simulink model "madar"  (Simulink 7.5)
settings: Solver=ode45  StartTime=0.0  StopTime=24  MaxStep=inf  RelTol=1e-3
values from neighbouring files (symbols this model uses):
  R1 = Req/2    [trans-test.m]
  R2 = (Req/2)*((Vlv/Vhv)^2)    [trans-test.m]
  Rc = Voc^2/Pc    [trans-test.m]
  S = input('enter the power')    [trans-test.m]
  Vhv = input('enter high voltage')    [trans-test.m]
  Vlv = input('enter low voltage')    [trans-test.m]
  X1 = Xeq/2    [trans-test.m]
  X2 = (Xeq/2)*((Vlv/Vhv)^2)    [trans-test.m]
  Xm = Voc/Im    [trans-test.m]
libraries: powerlib x23, powerlib_extras x6
settings Model: Creator=Kian  LastModifiedBy=Kian
settings SolverCC: AutoInsertRateTranBlk=on
settings DataIOCC: OutputSaveName=Iout
settings DebuggingCC: SolverPrmCheckMsg=none

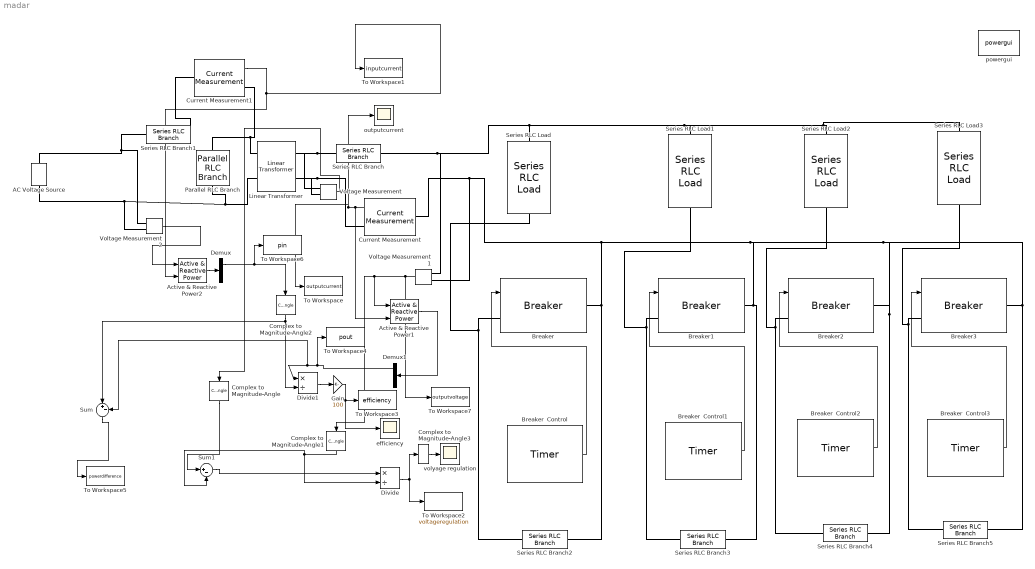
== system madar ==
  AC Voltage Source : powerlib/Electrical Sources/AC Voltage Source  DialogController=POWERSYS.PowerSysDialog  SystemSampleTime=-1  Amplitude=Vhv*(2^.5)  Phase=0  Frequency=50  SampleTime=0  Measurements=None
  Active & Reactive Power1 : powerlib_extras/Measurements/Active & Reactive Power  DialogController=POWERSYS.PowerSysDialog  SystemSampleTime=-1  f1=50
  Active & Reactive Power2 : powerlib_extras/Measurements/Active & Reactive Power  DialogController=POWERSYS.PowerSysDialog  SystemSampleTime=-1  f1=50
  Breaker{,1..3} (4 alike) : powerlib/Elements/Breaker  DialogController=POWERSYS.PowerSysDialog  SystemSampleTime=-1  BreakerResistance=0.000001  InitialState=0  SnubberResistance=inf  SnubberCapacitance=0  SwitchingTimes="[ 1/60  5/60 ]"  External=on  Measurements=None  MoreParameters=off  NoBreakLoop=off
  Breaker  Control : powerlib_extras/Control  Blocks/Timer  DialogController=POWERSYS.PowerSysDialog  SystemSampleTime=-1  t=[0 0.00001 7]  e=[0 1 0 ]
  Breaker  Control1 : powerlib_extras/Control  Blocks/Timer  DialogController=POWERSYS.PowerSysDialog  SystemSampleTime=-1  t=[0 7 12]  e=[0 1 0 ]
  Breaker  Control2 : powerlib_extras/Control  Blocks/Timer  DialogController=POWERSYS.PowerSysDialog  SystemSampleTime=-1  t=[0 12 20]  e=[0 1 0 ]
  Breaker  Control3 : powerlib_extras/Control  Blocks/Timer  DialogController=POWERSYS.PowerSysDialog  SystemSampleTime=-1  t=[0 20 24]  e=[0 1 0 ]
  Complex to Magnitude-Angle{,1..3} (4 alike) : ComplexToMagnitudeAngle  Output=Magnitude
  Current Measurement : powerlib/Measurements/Current Measurement  DialogController=POWERSYS.PowerSysDialog  SystemSampleTime=-1  PhasorSimulation=off  OutputType=Complex  PSBequivalent=0
  Current Measurement1 : powerlib/Measurements/Current Measurement  DialogController=POWERSYS.PowerSysDialog  SystemSampleTime=-1  PhasorSimulation=off  OutputType=Complex  PSBequivalent=0
  Demux : Demux  Outputs=2
  Demux1 : Demux  Outputs=2
  Divide : Product  Inputs=*/  OutDataType=fixdt(1, 16)  OutScaling=2^-10
  Divide1 : Product  Inputs=*/  OutDataType=fixdt(1, 16)  OutScaling=2^-10
  Gain : Gain  Gain=100  ParameterDataType=fixdt(1, 16)  ParameterScaling=2^0  OutDataType=fixdt(1, 16)  OutScaling=2^0
  Linear Transformer : powerlib/Elements/Linear Transformer  DialogController=POWERSYS.PowerSysDialog  PhysicalDomain=powersysdomain  SubClassName=unknown  LeftPortType=p1  RightPortType=p1  LConnTagsString=a|b  RConnTagsString=A|B  UNITS=SI  NominalPower=[ S 50 ]  winding1="[ Vhv  0  0 ]"  winding2="[ Vlv  0  0 ]"  ThreeWindings=off  winding3=[ ]  RmLm=[ 0 0 ]  Measurements=None  DataType=off
  Parallel RLC Branch : powerlib/Elements/Parallel RLC Branch  DialogController=POWERSYS.PowerSysDialog  PhysicalDomain=powersysdomain  SubClassName=unknown  LeftPortType=p1  RightPortType=p1  LConnTagsString=a  RConnTagsString=__new0  BranchType=RL  Resistance=Rc*((Vhv/Vlv)^2)  Inductance=Xm*((Vhv/Vlv)^2)/(100*pi)  SetiL0=off  InitialCurrent=0  Capacitance=0  Setx0=off  InitialVoltage=0  Measurements=None
  Series RLC Branch : powerlib/Elements/Series RLC Branch  DialogController=POWERSYS.PowerSysDialog  PhysicalDomain=powersysdomain  SubClassName=unknown  LeftPortType=p1  RightPortType=p1  LConnTagsString=__new0  RConnTagsString=__new0  BranchType=RL  Resistance=R2  Inductance=X2/(100*pi)  SetiL0=off  InitialCurrent=0  Capacitance=0  Setx0=off  InitialVoltage=0  Measurements=None
  Series RLC Branch1 : powerlib/Elements/Series RLC Branch  DialogController=POWERSYS.PowerSysDialog  PhysicalDomain=powersysdomain  SubClassName=unknown  LeftPortType=p1  RightPortType=p1  LConnTagsString=__new0  RConnTagsString=__new0  BranchType=RL  Resistance=R1  Inductance=X1/(100*pi)  SetiL0=off  InitialCurrent=0  Capacitance=0  Setx0=off  InitialVoltage=0  Measurements=None
  Series RLC Branch{2..5} (4 alike) : powerlib/Elements/Series RLC Branch  DialogController=POWERSYS.PowerSysDialog  PhysicalDomain=powersysdomain  SubClassName=unknown  LeftPortType=p1  RightPortType=p1  LConnTagsString=__new0  RConnTagsString=__new0  BranchType=R  Resistance=1000000  Inductance=X2/(100*pi)  SetiL0=off  InitialCurrent=0  Capacitance=0  Setx0=off  InitialVoltage=0  Measurements=None
  Series RLC Load : powerlib/Elements/Series RLC Load  DialogController=POWERSYS.PowerSysDialog  PhysicalDomain=powersysdomain  SubClassName=unknown  LeftPortType=p1  RightPortType=p1  LConnTagsString=a  RConnTagsString=__new0  NominalVoltage=Vlv  NominalFrequency=50  ActivePower=0.3*S*0.8  InductivePower=0.3*S*0.6  CapacitivePower=0  Setx0=off  InitialVoltage=0  SetiL0=off  InitialCurrent=0  Measurements=None
  Series RLC Load1 : powerlib/Elements/Series RLC Load  DialogController=POWERSYS.PowerSysDialog  PhysicalDomain=powersysdomain  SubClassName=unknown  LeftPortType=p1  RightPortType=p1  LConnTagsString=a  RConnTagsString=__new0  NominalVoltage=Vlv  NominalFrequency=50  ActivePower=0.75*S  InductivePower=0  CapacitivePower=0  Setx0=off  InitialVoltage=0  SetiL0=off  InitialCurrent=0  Measurements=None
  Series RLC Load2 : powerlib/Elements/Series RLC Load  DialogController=POWERSYS.PowerSysDialog  PhysicalDomain=powersysdomain  SubClassName=unknown  LeftPortType=p1  RightPortType=p1  LConnTagsString=a  RConnTagsString=__new0  NominalVoltage=Vlv  NominalFrequency=50  ActivePower=S*0.9  InductivePower=S*0.435  CapacitivePower=0  Setx0=off  InitialVoltage=0  SetiL0=off  InitialCurrent=0  Measurements=None
  Series RLC Load3 : powerlib/Elements/Series RLC Load  DialogController=POWERSYS.PowerSysDialog  PhysicalDomain=powersysdomain  SubClassName=unknown  LeftPortType=p1  RightPortType=p1  LConnTagsString=a  RConnTagsString=__new0  NominalVoltage=Vlv  NominalFrequency=50  ActivePower=0.5*S*0.85  InductivePower=0.5*S*0.526  CapacitivePower=0  Setx0=off  InitialVoltage=0  SetiL0=off  InitialCurrent=0  Measurements=None
  Sum : Sum  Inputs=|+-  OutDataType=fixdt(1, 16)  OutScaling=2^0
  Sum1 : Sum  Inputs=|+-  OutDataType=fixdt(1, 16)  OutScaling=2^0
  To Workspace : ToWorkspace  VariableName=outputcurrent  SampleTime=-1  SaveFormat=Structure With Time
  To Workspace1 : ToWorkspace  VariableName=inputcurrent  SampleTime=-1  SaveFormat=Structure
  To Workspace2 : ToWorkspace  VariableName=voltageregulation  SampleTime=-1  SaveFormat=Structure With Time
  To Workspace3 : ToWorkspace  VariableName=efficiency  SampleTime=-1  SaveFormat=Structure
  To Workspace4 : ToWorkspace  VariableName=pout  SampleTime=-1  SaveFormat=Structure
  To Workspace5 : ToWorkspace  VariableName=powerdifference  SampleTime=-1  SaveFormat=Structure
  To Workspace6 : ToWorkspace  VariableName=pin  SampleTime=-1  SaveFormat=Structure
  To Workspace7 : ToWorkspace  VariableName=outputvoltage  SampleTime=-1  SaveFormat=Structure With Time
  Voltage Measurement : powerlib/Measurements/Voltage Measurement  DialogController=POWERSYS.PowerSysDialog  SystemSampleTime=-1  PhasorSimulation=off  OutputType=Complex  PSBequivalent=0
  Voltage Measurement1 : powerlib/Measurements/Voltage Measurement  DialogController=POWERSYS.PowerSysDialog  SystemSampleTime=-1  PhasorSimulation=off  OutputType=Complex  PSBequivalent=0
  Voltage Measurement2 : powerlib/Measurements/Voltage Measurement  DialogController=POWERSYS.PowerSysDialog  SystemSampleTime=-1  PhasorSimulation=off  OutputType=Complex  PSBequivalent=0
  efficiency : Scope
  outputcurrent : Scope
  powergui : powerlib/powergui  Priority=1  SystemSampleTime=-1  SimulationMode=Discrete  SampleTime=50e-6  frequency=60  SPID=off  DisableSnubberDevices=off  DisableRonSwitches=off  DisableVfSwitches=off  SwTol=0  Interpol=off  frequencyindice=50  echomessages=off  HookPort=off  DisplayEquations=off  FunctionMessages=off  EnableUseOfTLC=off  x0status=blocks  RestoreLinks=warning  ResistiveCurrentMeasurement=off  Ylog=off  Xlog=on  ShowGrid=off  save=off  variable=ZData  ZoomFFT=off  StartTime=0.0  cycles=1  DisplayStyle=1  FreqAxis=off  MaxFrequency=1000  frequencyindicesteady=1  display=off  methode=off
  volyage regulation : Scope
      settings: SaveName=ScopeData2
  wires:
  Breaker  Control/1 -> Breaker/1
  Breaker  Control1/1 -> Breaker1/1
  Breaker  Control2/1 -> Breaker2/1
  Breaker  Control3/1 -> Breaker3/1
  Current Measurement/1 -> Active & Reactive Power1/2, To Workspace/1, outputcurrent/1
  Current Measurement1/1 -> Active & Reactive Power2/2, To Workspace1/1
  Voltage Measurement1/1 -> To Workspace7/1, Complex to Magnitude-Angle1/1, Active & Reactive Power1/1
  Sum1/1 -> Divide/1
  Divide/1 -> To Workspace2/1, Complex to Magnitude-Angle3/1
  Voltage Measurement2/1 -> Active & Reactive Power2/1
  Active & Reactive Power1/1 -> Demux1/1
  Divide1/1 -> Gain/1
  Voltage Measurement/1 -> Complex to Magnitude-Angle/1
  Complex to Magnitude-Angle/1 -> Sum1/1
  Complex to Magnitude-Angle1/1 -> Divide/2, Sum1/2
  Active & Reactive Power2/1 -> Demux/1
  Gain/1 -> To Workspace3/1, efficiency/1
  Demux/1 -> To Workspace6/1, Complex to Magnitude-Angle2/1
  Demux1/1 -> Divide1/1, Sum/2, To Workspace4/1
  Sum/1 -> To Workspace5/1
  Complex to Magnitude-Angle2/1 -> Divide1/2, Sum/1
  Complex to Magnitude-Angle3/1 -> volyage regulation/1
  connections:
  Linear Transformer/LConn2 -- Parallel RLC Branch/RConn1 -- AC Voltage Source/LConn1 -- Voltage Measurement2/LConn2
  Parallel RLC Branch/LConn1 -- Linear Transformer/LConn1 -- Current Measurement1/RConn1
  Series RLC Load/RConn1 -- Breaker/LConn1 -- Series RLC Branch2/LConn1
  Series RLC Load1/RConn1 -- Series RLC Branch3/LConn1 -- Breaker1/LConn1
  Series RLC Load2/RConn1 -- Series RLC Branch4/LConn1 -- Breaker2/LConn1
  Series RLC Load3/RConn1 -- Series RLC Branch5/LConn1 -- Breaker3/LConn1
  Linear Transformer/RConn2 -- Current Measurement/RConn1 -- Voltage Measurement/LConn2
  Series RLC Branch/RConn1 -- Series RLC Load1/LConn1 -- Series RLC Load2/LConn1 -- Series RLC Load3/LConn1 -- Series RLC Load/LConn1 -- Voltage Measurement1/LConn1
  Current Measurement/LConn1 -- Series RLC Branch2/RConn1 -- Breaker/RConn1 -- Series RLC Branch5/RConn1 -- Breaker3/RConn1 -- Series RLC Branch4/RConn1 -- Breaker2/RConn1 -- Series RLC Branch3/RConn1 -- Breaker1/RConn1 -- Voltage Measurement1/LConn2
  Current Measurement1/LConn1 -- Series RLC Branch1/RConn1
  Linear Transformer/RConn1 -- Series RLC Branch/LConn1 -- Voltage Measurement/LConn1
  Voltage Measurement2/LConn1 -- AC Voltage Source/RConn1 -- Series RLC Branch1/LConn1
